simulink model "untitled1"  (R2019b)
settings: Solver=VariableStepAuto  StartTime=0.0  StopTime=sim  RelTol=1e-3
values from neighbouring files (symbols this model uses):
  A = [0, 1;-f(1), -f(2)]    [init.m]
  b = [0; 1]    [init.m]
  cT = [0 1]    [init.m]
libraries: simulink x1, cstblocks x1

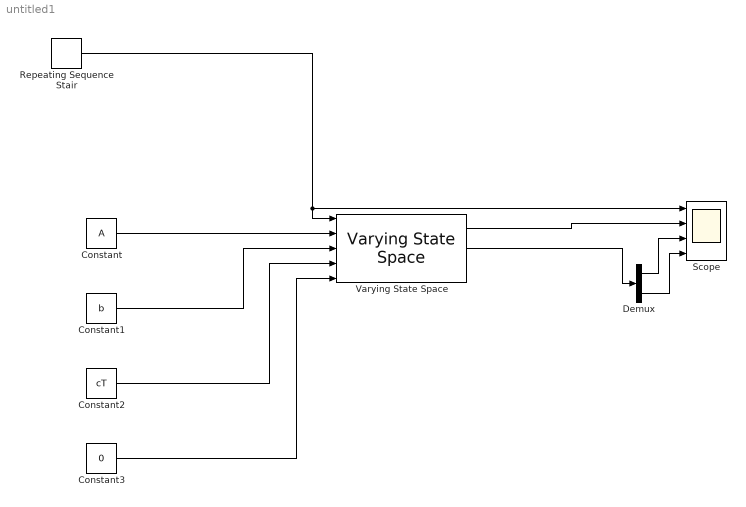
== system untitled1 ==
  Constant : Constant  Value=A  VectorParams1D=off
  Constant1 : Constant  Value=b  VectorParams1D=off
  Constant2 : Constant  Value=cT  VectorParams1D=off
  Constant3 : Constant  Value=0
  Demux : Demux  Outputs=2
  Repeating Sequence Stair : simulink/Sources/Repeating Sequence Stair  OutValues=data.Data  tsamp=-1  OutMin=[]  OutMax=[]  OutDataTypeStr=double  OutputDataTypeScalingMode=double  OutDataType=fixdt(0,8)  ConRadixGroup=Best Precision: Vector-wise  OutScaling=2^-12
  Scope : Scope  NumInputPorts=4
  Varying State Space : cstblocks/Linear Parameter Varying/Varying State Space  x0=0  xNames=''  OutputX=on  OutputDX=on
  wires:
  Constant/1 -> Varying State Space/2
  Constant1/1 -> Varying State Space/3
  Constant2/1 -> Varying State Space/4
  Constant3/1 -> Varying State Space/5
  Varying State Space/2 -> Demux/1
  Varying State Space/1 -> Scope/2
  Repeating Sequence Stair/1 -> Varying State Space/1, Scope/1
  Demux/1 -> Scope/3
  Demux/2 -> Scope/4
